simulink model "Ecm_2RC_battery"  (R2022a)
settings: Solver=FixedStepAuto  StartTime=0.0  StopTime=3600  FixedStep=0.1  RelTol=1e-3
values from neighbouring files (symbols this model uses):
  T_init = 293.15    [cell_data.mat]
libraries: fl_lib x1074, LiBatteryElements_lib x540, nesl_utility x102
(part 9 of 18)

== system Ecm_2RC_battery/Subsystem4/Subsystem4 ==
  Temp : Inport
  C1 : LiBatteryElements_lib/C_table  C_Table=C1_LUT F  SOC_Table=SOC_LUT  Temp_Table=Temperature_LUT K  v0=0 V
      settings: SourceProductBaseCode=SS  InternalSimscapePortConfiguration="{\"Bottom\":[],\"Left\":[{\"id\":\"p\",\"label\":\"+\",\"type\":\"foundation.electrical.electrical\"},{\"id\":\"T\",\"label\":\"T\",\"type\":\"input\"},{\"id\":\"SOC\",\"label\":\"SOC\",\"type\":\"input\"}],\"Right\":[{\"id\":\"n\",\"label\":\"-\",\"type\":\"foundation.electrical.electrical\"}],\"Top\":[]}"
  C2 : LiBatteryElements_lib/C_table  C_Table=C2_LUT F  SOC_Table=SOC_LUT  Temp_Table=Temperature_LUT K  v0=0 V
      settings: SourceProductBaseCode=SS  InternalSimscapePortConfiguration="{\"Bottom\":[],\"Left\":[{\"id\":\"p\",\"label\":\"+\",\"type\":\"foundation.electrical.electrical\"},{\"id\":\"T\",\"label\":\"T\",\"type\":\"input\"},{\"id\":\"SOC\",\"label\":\"SOC\",\"type\":\"input\"}],\"Right\":[{\"id\":\"n\",\"label\":\"-\",\"type\":\"foundation.electrical.electrical\"}],\"Top\":[]}"
  Controlled Temperature Source : fl_lib/Thermal/Thermal Sources/Controlled Temperature Source
      settings: SourceProductBaseCode=PW,SS,VE
  Convective Heat Transfer : fl_lib/Thermal/Thermal Elements/Convective Heat Transfer  area=cell_area m^2  heat_tr_coeff=h_conv W/(m^2 * K)  T_specify=off  T_priority=None  T=0 K  T_nominal_specify=off  T_nominal_unit=K  T_nominal_value=1  Q_specify=off  Q_priority=None  Q=0 W  Q_nominal_specify=off  Q_nominal_unit=W  Q_nominal_value=1
      settings: SourceProductBaseCode=PW,SS,VE
  Em_table : LiBatteryElements_lib/Em_table  C_Table=Capacity_LUT hr*A  Em_Table=Em_LUT V  SOC_Table=SOC_LUT  Temp_Table=Temperature_LUT K  Qinit=Qe_init hr*A
      settings: SourceProductBaseCode=SS  InternalSimscapePortConfiguration="{\"Bottom\":[],\"Left\":[{\"id\":\"p\",\"label\":\"+\",\"type\":\"foundation.electrical.electrical\"},{\"id\":\"C\",\"label\":\"C\",\"type\":\"output\"},{\"id\":\"SOC\",\"label\":\"SOC\",\"type\":\"output\"}],\"Right\":[{\"id\":\"n\",\"label\":\"-\",\"type\":\"foundation.electrical.electrical\"},{\"id\":\"T\",\"label\":\"T\",\"type\":\"input\"}],\"Top\":[]}"
  R0 : LiBatteryElements_lib/R_table  R_Table=R0_LUT Ohm  SOC_Table=SOC_LUT  Temp_Table=Temperature_LUT K
      settings: SourceProductBaseCode=SS  InternalSimscapePortConfiguration="{\"Bottom\":[],\"Left\":[{\"id\":\"p\",\"label\":\"+\",\"type\":\"foundation.electrical.electrical\"},{\"id\":\"T\",\"label\":\"T\",\"type\":\"input\"},{\"id\":\"SOC\",\"label\":\"SOC\",\"type\":\"input\"}],\"Right\":[{\"id\":\"n\",\"label\":\"-\",\"type\":\"foundation.electrical.electrical\"},{\"id\":\"pow\",\"label\":\"POW\",\"type\":\"output\"}],\"Top\":[]}"
  R1 : LiBatteryElements_lib/R_table  R_Table=R1_LUT Ohm  SOC_Table=SOC_LUT  Temp_Table=Temperature_LUT K
      settings: SourceProductBaseCode=SS  InternalSimscapePortConfiguration="{\"Bottom\":[],\"Left\":[{\"id\":\"p\",\"label\":\"+\",\"type\":\"foundation.electrical.electrical\"},{\"id\":\"T\",\"label\":\"T\",\"type\":\"input\"},{\"id\":\"SOC\",\"label\":\"SOC\",\"type\":\"input\"}],\"Right\":[{\"id\":\"n\",\"label\":\"-\",\"type\":\"foundation.electrical.electrical\"},{\"id\":\"pow\",\"label\":\"POW\",\"type\":\"output\"}],\"Top\":[]}"
  R2 : LiBatteryElements_lib/R_table  R_Table=R2_LUT Ohm  SOC_Table=SOC_LUT  Temp_Table=Temperature_LUT K
      settings: SourceProductBaseCode=SS  InternalSimscapePortConfiguration="{\"Bottom\":[],\"Left\":[{\"id\":\"p\",\"label\":\"+\",\"type\":\"foundation.electrical.electrical\"},{\"id\":\"T\",\"label\":\"T\",\"type\":\"input\"},{\"id\":\"SOC\",\"label\":\"SOC\",\"type\":\"input\"}],\"Right\":[{\"id\":\"n\",\"label\":\"-\",\"type\":\"foundation.electrical.electrical\"},{\"id\":\"pow\",\"label\":\"POW\",\"type\":\"output\"}],\"Top\":[]}"
  Simulink-PS Converter1 : nesl_utility/Simulink-PS Converter  PhysicalDomain=network_engine_domain  SubClassName=ps_input  LeftPortType=input  RightPortType=output  PseudoPeriodic=off  Frequencies=[]  NoiseDistribution=none  NoiseParameters=[]  Unit=degC  AffineConversion=on  FilteringAndDerivatives=zero  SimscapeFilterOrder=1  InputFilterTimeConstant=.001  UdotUserProvided=1
      settings: SourceProductBaseCode=SS,PW,VE
  Sum : Subsystem
      mask Display:
      | port_label('RConn',1,'+');
      | port_label('RConn',2,'+');
      | port_label('RConn',3,'+');
  Thermal Model : Subsystem
  Thermal Reference : fl_lib/Thermal/Thermal Elements/Thermal Reference
      settings: SourceProductBaseCode=PW,SS,VE
  + : PMIOPort  Side=Left
  SoC : PMIOPort  Port=2  Side=Right
  Charge : PMIOPort  Port=3  Side=Right
  - : PMIOPort  Port=4  Side=Right
  wires:
  Temp/1 -> Simulink-PS Converter1/1
  connections:
  C1/RConn1 -- R1/RConn1 -- R2/LConn1 -- C2/LConn1
  C1/LConn2 -- R0/LConn2 -- R2/LConn2 -- C2/LConn2 -- Thermal Model/RConn1 -- Em_table/RConn2 -- R1/LConn2
  R0/RConn2 -- Sum/RConn3
  R1/LConn1 -- C1/LConn1 -- Em_table/LConn1
  Convective Heat Transfer/RConn1 -- Thermal Model/LConn2
  R2/RConn1 -- R0/LConn1 -- C2/RConn1
  Sum/RConn2 -- R2/RConn2
  R1/RConn2 -- Sum/RConn1
  SoC/RConn1 -- R0/LConn3 -- C2/LConn3 -- R2/LConn3 -- Em_table/LConn3 -- C1/LConn3 -- R1/LConn3
  Sum/LConn1 -- Thermal Model/LConn1
  Controlled Temperature Source/RConn1 -- Simulink-PS Converter1/RConn1
  Thermal Reference/LConn1 -- Controlled Temperature Source/RConn2
  Controlled Temperature Source/LConn1 -- Convective Heat Transfer/LConn1
  Em_table/RConn1 -- -/RConn1
  R0/RConn1 -- +/RConn1
  Em_table/LConn2 -- Charge/RConn1

== system Ecm_2RC_battery/Subsystem4/Subsystem5 ==
  Temp : Inport
  C1 : LiBatteryElements_lib/C_table  C_Table=C1_LUT F  SOC_Table=SOC_LUT  Temp_Table=Temperature_LUT K  v0=0 V
      settings: SourceProductBaseCode=SS  InternalSimscapePortConfiguration="{\"Bottom\":[],\"Left\":[{\"id\":\"p\",\"label\":\"+\",\"type\":\"foundation.electrical.electrical\"},{\"id\":\"T\",\"label\":\"T\",\"type\":\"input\"},{\"id\":\"SOC\",\"label\":\"SOC\",\"type\":\"input\"}],\"Right\":[{\"id\":\"n\",\"label\":\"-\",\"type\":\"foundation.electrical.electrical\"}],\"Top\":[]}"
  C2 : LiBatteryElements_lib/C_table  C_Table=C2_LUT F  SOC_Table=SOC_LUT  Temp_Table=Temperature_LUT K  v0=0 V
      settings: SourceProductBaseCode=SS  InternalSimscapePortConfiguration="{\"Bottom\":[],\"Left\":[{\"id\":\"p\",\"label\":\"+\",\"type\":\"foundation.electrical.electrical\"},{\"id\":\"T\",\"label\":\"T\",\"type\":\"input\"},{\"id\":\"SOC\",\"label\":\"SOC\",\"type\":\"input\"}],\"Right\":[{\"id\":\"n\",\"label\":\"-\",\"type\":\"foundation.electrical.electrical\"}],\"Top\":[]}"
  Controlled Temperature Source : fl_lib/Thermal/Thermal Sources/Controlled Temperature Source
      settings: SourceProductBaseCode=PW,SS,VE
  Convective Heat Transfer : fl_lib/Thermal/Thermal Elements/Convective Heat Transfer  area=cell_area m^2  heat_tr_coeff=h_conv W/(m^2 * K)  T_specify=off  T_priority=None  T=0 K  T_nominal_specify=off  T_nominal_unit=K  T_nominal_value=1  Q_specify=off  Q_priority=None  Q=0 W  Q_nominal_specify=off  Q_nominal_unit=W  Q_nominal_value=1
      settings: SourceProductBaseCode=PW,SS,VE
  Em_table : LiBatteryElements_lib/Em_table  C_Table=Capacity_LUT hr*A  Em_Table=Em_LUT V  SOC_Table=SOC_LUT  Temp_Table=Temperature_LUT K  Qinit=Qe_init hr*A
      settings: SourceProductBaseCode=SS  InternalSimscapePortConfiguration="{\"Bottom\":[],\"Left\":[{\"id\":\"p\",\"label\":\"+\",\"type\":\"foundation.electrical.electrical\"},{\"id\":\"C\",\"label\":\"C\",\"type\":\"output\"},{\"id\":\"SOC\",\"label\":\"SOC\",\"type\":\"output\"}],\"Right\":[{\"id\":\"n\",\"label\":\"-\",\"type\":\"foundation.electrical.electrical\"},{\"id\":\"T\",\"label\":\"T\",\"type\":\"input\"}],\"Top\":[]}"
  R0 : LiBatteryElements_lib/R_table  R_Table=R0_LUT Ohm  SOC_Table=SOC_LUT  Temp_Table=Temperature_LUT K
      settings: SourceProductBaseCode=SS  InternalSimscapePortConfiguration="{\"Bottom\":[],\"Left\":[{\"id\":\"p\",\"label\":\"+\",\"type\":\"foundation.electrical.electrical\"},{\"id\":\"T\",\"label\":\"T\",\"type\":\"input\"},{\"id\":\"SOC\",\"label\":\"SOC\",\"type\":\"input\"}],\"Right\":[{\"id\":\"n\",\"label\":\"-\",\"type\":\"foundation.electrical.electrical\"},{\"id\":\"pow\",\"label\":\"POW\",\"type\":\"output\"}],\"Top\":[]}"
  R1 : LiBatteryElements_lib/R_table  R_Table=R1_LUT Ohm  SOC_Table=SOC_LUT  Temp_Table=Temperature_LUT K
      settings: SourceProductBaseCode=SS  InternalSimscapePortConfiguration="{\"Bottom\":[],\"Left\":[{\"id\":\"p\",\"label\":\"+\",\"type\":\"foundation.electrical.electrical\"},{\"id\":\"T\",\"label\":\"T\",\"type\":\"input\"},{\"id\":\"SOC\",\"label\":\"SOC\",\"type\":\"input\"}],\"Right\":[{\"id\":\"n\",\"label\":\"-\",\"type\":\"foundation.electrical.electrical\"},{\"id\":\"pow\",\"label\":\"POW\",\"type\":\"output\"}],\"Top\":[]}"
  R2 : LiBatteryElements_lib/R_table  R_Table=R2_LUT Ohm  SOC_Table=SOC_LUT  Temp_Table=Temperature_LUT K
      settings: SourceProductBaseCode=SS  InternalSimscapePortConfiguration="{\"Bottom\":[],\"Left\":[{\"id\":\"p\",\"label\":\"+\",\"type\":\"foundation.electrical.electrical\"},{\"id\":\"T\",\"label\":\"T\",\"type\":\"input\"},{\"id\":\"SOC\",\"label\":\"SOC\",\"type\":\"input\"}],\"Right\":[{\"id\":\"n\",\"label\":\"-\",\"type\":\"foundation.electrical.electrical\"},{\"id\":\"pow\",\"label\":\"POW\",\"type\":\"output\"}],\"Top\":[]}"
  Simulink-PS Converter1 : nesl_utility/Simulink-PS Converter  PhysicalDomain=network_engine_domain  SubClassName=ps_input  LeftPortType=input  RightPortType=output  PseudoPeriodic=off  Frequencies=[]  NoiseDistribution=none  NoiseParameters=[]  Unit=degC  AffineConversion=on  FilteringAndDerivatives=zero  SimscapeFilterOrder=1  InputFilterTimeConstant=.001  UdotUserProvided=1
      settings: SourceProductBaseCode=SS,PW,VE
  Sum : Subsystem
      mask Display:
      | port_label('RConn',1,'+');
      | port_label('RConn',2,'+');
      | port_label('RConn',3,'+');
  Thermal Model : Subsystem
  Thermal Reference : fl_lib/Thermal/Thermal Elements/Thermal Reference
      settings: SourceProductBaseCode=PW,SS,VE
  + : PMIOPort  Side=Left
  SoC : PMIOPort  Port=2  Side=Right
  Charge : PMIOPort  Port=3  Side=Right
  - : PMIOPort  Port=4  Side=Right
  wires:
  Temp/1 -> Simulink-PS Converter1/1
  connections:
  C1/RConn1 -- R1/RConn1 -- R2/LConn1 -- C2/LConn1
  C1/LConn2 -- R0/LConn2 -- R2/LConn2 -- C2/LConn2 -- Thermal Model/RConn1 -- Em_table/RConn2 -- R1/LConn2
  R0/RConn2 -- Sum/RConn3
  R1/LConn1 -- C1/LConn1 -- Em_table/LConn1
  Convective Heat Transfer/RConn1 -- Thermal Model/LConn2
  R2/RConn1 -- R0/LConn1 -- C2/RConn1
  Sum/RConn2 -- R2/RConn2
  R1/RConn2 -- Sum/RConn1
  SoC/RConn1 -- R0/LConn3 -- C2/LConn3 -- R2/LConn3 -- Em_table/LConn3 -- C1/LConn3 -- R1/LConn3
  Sum/LConn1 -- Thermal Model/LConn1
  Controlled Temperature Source/RConn1 -- Simulink-PS Converter1/RConn1
  Thermal Reference/LConn1 -- Controlled Temperature Source/RConn2
  Controlled Temperature Source/LConn1 -- Convective Heat Transfer/LConn1
  Em_table/RConn1 -- -/RConn1
  R0/RConn1 -- +/RConn1
  Em_table/LConn2 -- Charge/RConn1

== system Ecm_2RC_battery/Subsystem4/Subsystem6 ==
  Temp : Inport
  C1 : LiBatteryElements_lib/C_table  C_Table=C1_LUT F  SOC_Table=SOC_LUT  Temp_Table=Temperature_LUT K  v0=0 V
      settings: SourceProductBaseCode=SS  InternalSimscapePortConfiguration="{\"Bottom\":[],\"Left\":[{\"id\":\"p\",\"label\":\"+\",\"type\":\"foundation.electrical.electrical\"},{\"id\":\"T\",\"label\":\"T\",\"type\":\"input\"},{\"id\":\"SOC\",\"label\":\"SOC\",\"type\":\"input\"}],\"Right\":[{\"id\":\"n\",\"label\":\"-\",\"type\":\"foundation.electrical.electrical\"}],\"Top\":[]}"
  C2 : LiBatteryElements_lib/C_table  C_Table=C2_LUT F  SOC_Table=SOC_LUT  Temp_Table=Temperature_LUT K  v0=0 V
      settings: SourceProductBaseCode=SS  InternalSimscapePortConfiguration="{\"Bottom\":[],\"Left\":[{\"id\":\"p\",\"label\":\"+\",\"type\":\"foundation.electrical.electrical\"},{\"id\":\"T\",\"label\":\"T\",\"type\":\"input\"},{\"id\":\"SOC\",\"label\":\"SOC\",\"type\":\"input\"}],\"Right\":[{\"id\":\"n\",\"label\":\"-\",\"type\":\"foundation.electrical.electrical\"}],\"Top\":[]}"
  Controlled Temperature Source : fl_lib/Thermal/Thermal Sources/Controlled Temperature Source
      settings: SourceProductBaseCode=PW,SS,VE
  Convective Heat Transfer : fl_lib/Thermal/Thermal Elements/Convective Heat Transfer  area=cell_area m^2  heat_tr_coeff=h_conv W/(m^2 * K)  T_specify=off  T_priority=None  T=0 K  T_nominal_specify=off  T_nominal_unit=K  T_nominal_value=1  Q_specify=off  Q_priority=None  Q=0 W  Q_nominal_specify=off  Q_nominal_unit=W  Q_nominal_value=1
      settings: SourceProductBaseCode=PW,SS,VE
  Em_table : LiBatteryElements_lib/Em_table  C_Table=Capacity_LUT hr*A  Em_Table=Em_LUT V  SOC_Table=SOC_LUT  Temp_Table=Temperature_LUT K  Qinit=Qe_init hr*A
      settings: SourceProductBaseCode=SS  InternalSimscapePortConfiguration="{\"Bottom\":[],\"Left\":[{\"id\":\"p\",\"label\":\"+\",\"type\":\"foundation.electrical.electrical\"},{\"id\":\"C\",\"label\":\"C\",\"type\":\"output\"},{\"id\":\"SOC\",\"label\":\"SOC\",\"type\":\"output\"}],\"Right\":[{\"id\":\"n\",\"label\":\"-\",\"type\":\"foundation.electrical.electrical\"},{\"id\":\"T\",\"label\":\"T\",\"type\":\"input\"}],\"Top\":[]}"
  R0 : LiBatteryElements_lib/R_table  R_Table=R0_LUT Ohm  SOC_Table=SOC_LUT  Temp_Table=Temperature_LUT K
      settings: SourceProductBaseCode=SS  InternalSimscapePortConfiguration="{\"Bottom\":[],\"Left\":[{\"id\":\"p\",\"label\":\"+\",\"type\":\"foundation.electrical.electrical\"},{\"id\":\"T\",\"label\":\"T\",\"type\":\"input\"},{\"id\":\"SOC\",\"label\":\"SOC\",\"type\":\"input\"}],\"Right\":[{\"id\":\"n\",\"label\":\"-\",\"type\":\"foundation.electrical.electrical\"},{\"id\":\"pow\",\"label\":\"POW\",\"type\":\"output\"}],\"Top\":[]}"
  R1 : LiBatteryElements_lib/R_table  R_Table=R1_LUT Ohm  SOC_Table=SOC_LUT  Temp_Table=Temperature_LUT K
      settings: SourceProductBaseCode=SS  InternalSimscapePortConfiguration="{\"Bottom\":[],\"Left\":[{\"id\":\"p\",\"label\":\"+\",\"type\":\"foundation.electrical.electrical\"},{\"id\":\"T\",\"label\":\"T\",\"type\":\"input\"},{\"id\":\"SOC\",\"label\":\"SOC\",\"type\":\"input\"}],\"Right\":[{\"id\":\"n\",\"label\":\"-\",\"type\":\"foundation.electrical.electrical\"},{\"id\":\"pow\",\"label\":\"POW\",\"type\":\"output\"}],\"Top\":[]}"
  R2 : LiBatteryElements_lib/R_table  R_Table=R2_LUT Ohm  SOC_Table=SOC_LUT  Temp_Table=Temperature_LUT K
      settings: SourceProductBaseCode=SS  InternalSimscapePortConfiguration="{\"Bottom\":[],\"Left\":[{\"id\":\"p\",\"label\":\"+\",\"type\":\"foundation.electrical.electrical\"},{\"id\":\"T\",\"label\":\"T\",\"type\":\"input\"},{\"id\":\"SOC\",\"label\":\"SOC\",\"type\":\"input\"}],\"Right\":[{\"id\":\"n\",\"label\":\"-\",\"type\":\"foundation.electrical.electrical\"},{\"id\":\"pow\",\"label\":\"POW\",\"type\":\"output\"}],\"Top\":[]}"
  Simulink-PS Converter1 : nesl_utility/Simulink-PS Converter  PhysicalDomain=network_engine_domain  SubClassName=ps_input  LeftPortType=input  RightPortType=output  PseudoPeriodic=off  Frequencies=[]  NoiseDistribution=none  NoiseParameters=[]  Unit=degC  AffineConversion=on  FilteringAndDerivatives=zero  SimscapeFilterOrder=1  InputFilterTimeConstant=.001  UdotUserProvided=1
      settings: SourceProductBaseCode=SS,PW,VE
  Sum : Subsystem
      mask Display:
      | port_label('RConn',1,'+');
      | port_label('RConn',2,'+');
      | port_label('RConn',3,'+');
  Thermal Model : Subsystem
  Thermal Reference : fl_lib/Thermal/Thermal Elements/Thermal Reference
      settings: SourceProductBaseCode=PW,SS,VE
  + : PMIOPort  Side=Left
  SoC : PMIOPort  Port=2  Side=Right
  Charge : PMIOPort  Port=3  Side=Right
  - : PMIOPort  Port=4  Side=Right
  wires:
  Temp/1 -> Simulink-PS Converter1/1
  connections:
  C1/RConn1 -- R1/RConn1 -- R2/LConn1 -- C2/LConn1
  C1/LConn2 -- R0/LConn2 -- R2/LConn2 -- C2/LConn2 -- Thermal Model/RConn1 -- Em_table/RConn2 -- R1/LConn2
  R0/RConn2 -- Sum/RConn3
  R1/LConn1 -- C1/LConn1 -- Em_table/LConn1
  Convective Heat Transfer/RConn1 -- Thermal Model/LConn2
  R2/RConn1 -- R0/LConn1 -- C2/RConn1
  Sum/RConn2 -- R2/RConn2
  R1/RConn2 -- Sum/RConn1
  SoC/RConn1 -- R0/LConn3 -- C2/LConn3 -- R2/LConn3 -- Em_table/LConn3 -- C1/LConn3 -- R1/LConn3
  Sum/LConn1 -- Thermal Model/LConn1
  Controlled Temperature Source/RConn1 -- Simulink-PS Converter1/RConn1
  Thermal Reference/LConn1 -- Controlled Temperature Source/RConn2
  Controlled Temperature Source/LConn1 -- Convective Heat Transfer/LConn1
  Em_table/RConn1 -- -/RConn1
  R0/RConn1 -- +/RConn1
  Em_table/LConn2 -- Charge/RConn1

== system Ecm_2RC_battery/Subsystem4/Subsystem7 ==
  Temp : Inport
  C1 : LiBatteryElements_lib/C_table  C_Table=C1_LUT F  SOC_Table=SOC_LUT  Temp_Table=Temperature_LUT K  v0=0 V
      settings: SourceProductBaseCode=SS  InternalSimscapePortConfiguration="{\"Bottom\":[],\"Left\":[{\"id\":\"p\",\"label\":\"+\",\"type\":\"foundation.electrical.electrical\"},{\"id\":\"T\",\"label\":\"T\",\"type\":\"input\"},{\"id\":\"SOC\",\"label\":\"SOC\",\"type\":\"input\"}],\"Right\":[{\"id\":\"n\",\"label\":\"-\",\"type\":\"foundation.electrical.electrical\"}],\"Top\":[]}"
  C2 : LiBatteryElements_lib/C_table  C_Table=C2_LUT F  SOC_Table=SOC_LUT  Temp_Table=Temperature_LUT K  v0=0 V
      settings: SourceProductBaseCode=SS  InternalSimscapePortConfiguration="{\"Bottom\":[],\"Left\":[{\"id\":\"p\",\"label\":\"+\",\"type\":\"foundation.electrical.electrical\"},{\"id\":\"T\",\"label\":\"T\",\"type\":\"input\"},{\"id\":\"SOC\",\"label\":\"SOC\",\"type\":\"input\"}],\"Right\":[{\"id\":\"n\",\"label\":\"-\",\"type\":\"foundation.electrical.electrical\"}],\"Top\":[]}"
  Controlled Temperature Source : fl_lib/Thermal/Thermal Sources/Controlled Temperature Source
      settings: SourceProductBaseCode=PW,SS,VE
  Convective Heat Transfer : fl_lib/Thermal/Thermal Elements/Convective Heat Transfer  area=cell_area m^2  heat_tr_coeff=h_conv W/(m^2 * K)  T_specify=off  T_priority=None  T=0 K  T_nominal_specify=off  T_nominal_unit=K  T_nominal_value=1  Q_specify=off  Q_priority=None  Q=0 W  Q_nominal_specify=off  Q_nominal_unit=W  Q_nominal_value=1
      settings: SourceProductBaseCode=PW,SS,VE
  Em_table : LiBatteryElements_lib/Em_table  C_Table=Capacity_LUT hr*A  Em_Table=Em_LUT V  SOC_Table=SOC_LUT  Temp_Table=Temperature_LUT K  Qinit=Qe_init hr*A
      settings: SourceProductBaseCode=SS  InternalSimscapePortConfiguration="{\"Bottom\":[],\"Left\":[{\"id\":\"p\",\"label\":\"+\",\"type\":\"foundation.electrical.electrical\"},{\"id\":\"C\",\"label\":\"C\",\"type\":\"output\"},{\"id\":\"SOC\",\"label\":\"SOC\",\"type\":\"output\"}],\"Right\":[{\"id\":\"n\",\"label\":\"-\",\"type\":\"foundation.electrical.electrical\"},{\"id\":\"T\",\"label\":\"T\",\"type\":\"input\"}],\"Top\":[]}"
  R0 : LiBatteryElements_lib/R_table  R_Table=R0_LUT Ohm  SOC_Table=SOC_LUT  Temp_Table=Temperature_LUT K
      settings: SourceProductBaseCode=SS  InternalSimscapePortConfiguration="{\"Bottom\":[],\"Left\":[{\"id\":\"p\",\"label\":\"+\",\"type\":\"foundation.electrical.electrical\"},{\"id\":\"T\",\"label\":\"T\",\"type\":\"input\"},{\"id\":\"SOC\",\"label\":\"SOC\",\"type\":\"input\"}],\"Right\":[{\"id\":\"n\",\"label\":\"-\",\"type\":\"foundation.electrical.electrical\"},{\"id\":\"pow\",\"label\":\"POW\",\"type\":\"output\"}],\"Top\":[]}"
  R1 : LiBatteryElements_lib/R_table  R_Table=R1_LUT Ohm  SOC_Table=SOC_LUT  Temp_Table=Temperature_LUT K
      settings: SourceProductBaseCode=SS  InternalSimscapePortConfiguration="{\"Bottom\":[],\"Left\":[{\"id\":\"p\",\"label\":\"+\",\"type\":\"foundation.electrical.electrical\"},{\"id\":\"T\",\"label\":\"T\",\"type\":\"input\"},{\"id\":\"SOC\",\"label\":\"SOC\",\"type\":\"input\"}],\"Right\":[{\"id\":\"n\",\"label\":\"-\",\"type\":\"foundation.electrical.electrical\"},{\"id\":\"pow\",\"label\":\"POW\",\"type\":\"output\"}],\"Top\":[]}"
  R2 : LiBatteryElements_lib/R_table  R_Table=R2_LUT Ohm  SOC_Table=SOC_LUT  Temp_Table=Temperature_LUT K
      settings: SourceProductBaseCode=SS  InternalSimscapePortConfiguration="{\"Bottom\":[],\"Left\":[{\"id\":\"p\",\"label\":\"+\",\"type\":\"foundation.electrical.electrical\"},{\"id\":\"T\",\"label\":\"T\",\"type\":\"input\"},{\"id\":\"SOC\",\"label\":\"SOC\",\"type\":\"input\"}],\"Right\":[{\"id\":\"n\",\"label\":\"-\",\"type\":\"foundation.electrical.electrical\"},{\"id\":\"pow\",\"label\":\"POW\",\"type\":\"output\"}],\"Top\":[]}"
  Simulink-PS Converter1 : nesl_utility/Simulink-PS Converter  PhysicalDomain=network_engine_domain  SubClassName=ps_input  LeftPortType=input  RightPortType=output  PseudoPeriodic=off  Frequencies=[]  NoiseDistribution=none  NoiseParameters=[]  Unit=degC  AffineConversion=on  FilteringAndDerivatives=zero  SimscapeFilterOrder=1  InputFilterTimeConstant=.001  UdotUserProvided=1
      settings: SourceProductBaseCode=SS,PW,VE
  Sum : Subsystem
      mask Display:
      | port_label('RConn',1,'+');
      | port_label('RConn',2,'+');
      | port_label('RConn',3,'+');
  Thermal Model : Subsystem
  Thermal Reference : fl_lib/Thermal/Thermal Elements/Thermal Reference
      settings: SourceProductBaseCode=PW,SS,VE
  + : PMIOPort  Side=Left
  SoC : PMIOPort  Port=2  Side=Right
  Charge : PMIOPort  Port=3  Side=Right
  - : PMIOPort  Port=4  Side=Right
  wires:
  Temp/1 -> Simulink-PS Converter1/1
  connections:
  C1/RConn1 -- R1/RConn1 -- R2/LConn1 -- C2/LConn1
  C1/LConn2 -- R0/LConn2 -- R2/LConn2 -- C2/LConn2 -- Thermal Model/RConn1 -- Em_table/RConn2 -- R1/LConn2
  R0/RConn2 -- Sum/RConn3
  R1/LConn1 -- C1/LConn1 -- Em_table/LConn1
  Convective Heat Transfer/RConn1 -- Thermal Model/LConn2
  R2/RConn1 -- R0/LConn1 -- C2/RConn1
  Sum/RConn2 -- R2/RConn2
  R1/RConn2 -- Sum/RConn1
  SoC/RConn1 -- R0/LConn3 -- C2/LConn3 -- R2/LConn3 -- Em_table/LConn3 -- C1/LConn3 -- R1/LConn3
  Sum/LConn1 -- Thermal Model/LConn1
  Controlled Temperature Source/RConn1 -- Simulink-PS Converter1/RConn1
  Thermal Reference/LConn1 -- Controlled Temperature Source/RConn2
  Controlled Temperature Source/LConn1 -- Convective Heat Transfer/LConn1
  Em_table/RConn1 -- -/RConn1
  R0/RConn1 -- +/RConn1
  Em_table/LConn2 -- Charge/RConn1

== system Ecm_2RC_battery/Subsystem4/Subsystem8 ==
  Temp : Inport
  C1 : LiBatteryElements_lib/C_table  C_Table=C1_LUT F  SOC_Table=SOC_LUT  Temp_Table=Temperature_LUT K  v0=0 V
      settings: SourceProductBaseCode=SS  InternalSimscapePortConfiguration="{\"Bottom\":[],\"Left\":[{\"id\":\"p\",\"label\":\"+\",\"type\":\"foundation.electrical.electrical\"},{\"id\":\"T\",\"label\":\"T\",\"type\":\"input\"},{\"id\":\"SOC\",\"label\":\"SOC\",\"type\":\"input\"}],\"Right\":[{\"id\":\"n\",\"label\":\"-\",\"type\":\"foundation.electrical.electrical\"}],\"Top\":[]}"
  C2 : LiBatteryElements_lib/C_table  C_Table=C2_LUT F  SOC_Table=SOC_LUT  Temp_Table=Temperature_LUT K  v0=0 V
      settings: SourceProductBaseCode=SS  InternalSimscapePortConfiguration="{\"Bottom\":[],\"Left\":[{\"id\":\"p\",\"label\":\"+\",\"type\":\"foundation.electrical.electrical\"},{\"id\":\"T\",\"label\":\"T\",\"type\":\"input\"},{\"id\":\"SOC\",\"label\":\"SOC\",\"type\":\"input\"}],\"Right\":[{\"id\":\"n\",\"label\":\"-\",\"type\":\"foundation.electrical.electrical\"}],\"Top\":[]}"
  Controlled Temperature Source : fl_lib/Thermal/Thermal Sources/Controlled Temperature Source
      settings: SourceProductBaseCode=PW,SS,VE
  Convective Heat Transfer : fl_lib/Thermal/Thermal Elements/Convective Heat Transfer  area=cell_area m^2  heat_tr_coeff=h_conv W/(m^2 * K)  T_specify=off  T_priority=None  T=0 K  T_nominal_specify=off  T_nominal_unit=K  T_nominal_value=1  Q_specify=off  Q_priority=None  Q=0 W  Q_nominal_specify=off  Q_nominal_unit=W  Q_nominal_value=1
      settings: SourceProductBaseCode=PW,SS,VE
  Em_table : LiBatteryElements_lib/Em_table  C_Table=Capacity_LUT hr*A  Em_Table=Em_LUT V  SOC_Table=SOC_LUT  Temp_Table=Temperature_LUT K  Qinit=Qe_init hr*A
      settings: SourceProductBaseCode=SS  InternalSimscapePortConfiguration="{\"Bottom\":[],\"Left\":[{\"id\":\"p\",\"label\":\"+\",\"type\":\"foundation.electrical.electrical\"},{\"id\":\"C\",\"label\":\"C\",\"type\":\"output\"},{\"id\":\"SOC\",\"label\":\"SOC\",\"type\":\"output\"}],\"Right\":[{\"id\":\"n\",\"label\":\"-\",\"type\":\"foundation.electrical.electrical\"},{\"id\":\"T\",\"label\":\"T\",\"type\":\"input\"}],\"Top\":[]}"
  R0 : LiBatteryElements_lib/R_table  R_Table=R0_LUT Ohm  SOC_Table=SOC_LUT  Temp_Table=Temperature_LUT K
      settings: SourceProductBaseCode=SS  InternalSimscapePortConfiguration="{\"Bottom\":[],\"Left\":[{\"id\":\"p\",\"label\":\"+\",\"type\":\"foundation.electrical.electrical\"},{\"id\":\"T\",\"label\":\"T\",\"type\":\"input\"},{\"id\":\"SOC\",\"label\":\"SOC\",\"type\":\"input\"}],\"Right\":[{\"id\":\"n\",\"label\":\"-\",\"type\":\"foundation.electrical.electrical\"},{\"id\":\"pow\",\"label\":\"POW\",\"type\":\"output\"}],\"Top\":[]}"
  R1 : LiBatteryElements_lib/R_table  R_Table=R1_LUT Ohm  SOC_Table=SOC_LUT  Temp_Table=Temperature_LUT K
      settings: SourceProductBaseCode=SS  InternalSimscapePortConfiguration="{\"Bottom\":[],\"Left\":[{\"id\":\"p\",\"label\":\"+\",\"type\":\"foundation.electrical.electrical\"},{\"id\":\"T\",\"label\":\"T\",\"type\":\"input\"},{\"id\":\"SOC\",\"label\":\"SOC\",\"type\":\"input\"}],\"Right\":[{\"id\":\"n\",\"label\":\"-\",\"type\":\"foundation.electrical.electrical\"},{\"id\":\"pow\",\"label\":\"POW\",\"type\":\"output\"}],\"Top\":[]}"
  R2 : LiBatteryElements_lib/R_table  R_Table=R2_LUT Ohm  SOC_Table=SOC_LUT  Temp_Table=Temperature_LUT K
      settings: SourceProductBaseCode=SS  InternalSimscapePortConfiguration="{\"Bottom\":[],\"Left\":[{\"id\":\"p\",\"label\":\"+\",\"type\":\"foundation.electrical.electrical\"},{\"id\":\"T\",\"label\":\"T\",\"type\":\"input\"},{\"id\":\"SOC\",\"label\":\"SOC\",\"type\":\"input\"}],\"Right\":[{\"id\":\"n\",\"label\":\"-\",\"type\":\"foundation.electrical.electrical\"},{\"id\":\"pow\",\"label\":\"POW\",\"type\":\"output\"}],\"Top\":[]}"
  Simulink-PS Converter1 : nesl_utility/Simulink-PS Converter  PhysicalDomain=network_engine_domain  SubClassName=ps_input  LeftPortType=input  RightPortType=output  PseudoPeriodic=off  Frequencies=[]  NoiseDistribution=none  NoiseParameters=[]  Unit=degC  AffineConversion=on  FilteringAndDerivatives=zero  SimscapeFilterOrder=1  InputFilterTimeConstant=.001  UdotUserProvided=1
      settings: SourceProductBaseCode=SS,PW,VE
  Sum : Subsystem
      mask Display:
      | port_label('RConn',1,'+');
      | port_label('RConn',2,'+');
      | port_label('RConn',3,'+');
  Thermal Model : Subsystem
  Thermal Reference : fl_lib/Thermal/Thermal Elements/Thermal Reference
      settings: SourceProductBaseCode=PW,SS,VE
  + : PMIOPort  Side=Left
  SoC : PMIOPort  Port=2  Side=Right
  Charge : PMIOPort  Port=3  Side=Right
  - : PMIOPort  Port=4  Side=Right
  wires:
  Temp/1 -> Simulink-PS Converter1/1
  connections:
  C1/RConn1 -- R1/RConn1 -- R2/LConn1 -- C2/LConn1
  C1/LConn2 -- R0/LConn2 -- R2/LConn2 -- C2/LConn2 -- Thermal Model/RConn1 -- Em_table/RConn2 -- R1/LConn2
  R0/RConn2 -- Sum/RConn3
  R1/LConn1 -- C1/LConn1 -- Em_table/LConn1
  Convective Heat Transfer/RConn1 -- Thermal Model/LConn2
  R2/RConn1 -- R0/LConn1 -- C2/RConn1
  Sum/RConn2 -- R2/RConn2
  R1/RConn2 -- Sum/RConn1
  SoC/RConn1 -- R0/LConn3 -- C2/LConn3 -- R2/LConn3 -- Em_table/LConn3 -- C1/LConn3 -- R1/LConn3
  Sum/LConn1 -- Thermal Model/LConn1
  Controlled Temperature Source/RConn1 -- Simulink-PS Converter1/RConn1
  Thermal Reference/LConn1 -- Controlled Temperature Source/RConn2
  Controlled Temperature Source/LConn1 -- Convective Heat Transfer/LConn1
  Em_table/RConn1 -- -/RConn1
  R0/RConn1 -- +/RConn1
  Em_table/LConn2 -- Charge/RConn1

== system Ecm_2RC_battery/Subsystem4/Subsystem9 ==
  Temp : Inport
  C1 : LiBatteryElements_lib/C_table  C_Table=C1_LUT F  SOC_Table=SOC_LUT  Temp_Table=Temperature_LUT K  v0=0 V
      settings: SourceProductBaseCode=SS  InternalSimscapePortConfiguration="{\"Bottom\":[],\"Left\":[{\"id\":\"p\",\"label\":\"+\",\"type\":\"foundation.electrical.electrical\"},{\"id\":\"T\",\"label\":\"T\",\"type\":\"input\"},{\"id\":\"SOC\",\"label\":\"SOC\",\"type\":\"input\"}],\"Right\":[{\"id\":\"n\",\"label\":\"-\",\"type\":\"foundation.electrical.electrical\"}],\"Top\":[]}"
  C2 : LiBatteryElements_lib/C_table  C_Table=C2_LUT F  SOC_Table=SOC_LUT  Temp_Table=Temperature_LUT K  v0=0 V
      settings: SourceProductBaseCode=SS  InternalSimscapePortConfiguration="{\"Bottom\":[],\"Left\":[{\"id\":\"p\",\"label\":\"+\",\"type\":\"foundation.electrical.electrical\"},{\"id\":\"T\",\"label\":\"T\",\"type\":\"input\"},{\"id\":\"SOC\",\"label\":\"SOC\",\"type\":\"input\"}],\"Right\":[{\"id\":\"n\",\"label\":\"-\",\"type\":\"foundation.electrical.electrical\"}],\"Top\":[]}"
  Controlled Temperature Source : fl_lib/Thermal/Thermal Sources/Controlled Temperature Source
      settings: SourceProductBaseCode=PW,SS,VE
  Convective Heat Transfer : fl_lib/Thermal/Thermal Elements/Convective Heat Transfer  area=cell_area m^2  heat_tr_coeff=h_conv W/(m^2 * K)  T_specify=off  T_priority=None  T=0 K  T_nominal_specify=off  T_nominal_unit=K  T_nominal_value=1  Q_specify=off  Q_priority=None  Q=0 W  Q_nominal_specify=off  Q_nominal_unit=W  Q_nominal_value=1
      settings: SourceProductBaseCode=PW,SS,VE
  Em_table : LiBatteryElements_lib/Em_table  C_Table=Capacity_LUT hr*A  Em_Table=Em_LUT V  SOC_Table=SOC_LUT  Temp_Table=Temperature_LUT K  Qinit=Qe_init hr*A
      settings: SourceProductBaseCode=SS  InternalSimscapePortConfiguration="{\"Bottom\":[],\"Left\":[{\"id\":\"p\",\"label\":\"+\",\"type\":\"foundation.electrical.electrical\"},{\"id\":\"C\",\"label\":\"C\",\"type\":\"output\"},{\"id\":\"SOC\",\"label\":\"SOC\",\"type\":\"output\"}],\"Right\":[{\"id\":\"n\",\"label\":\"-\",\"type\":\"foundation.electrical.electrical\"},{\"id\":\"T\",\"label\":\"T\",\"type\":\"input\"}],\"Top\":[]}"
  R0 : LiBatteryElements_lib/R_table  R_Table=R0_LUT Ohm  SOC_Table=SOC_LUT  Temp_Table=Temperature_LUT K
      settings: SourceProductBaseCode=SS  InternalSimscapePortConfiguration="{\"Bottom\":[],\"Left\":[{\"id\":\"p\",\"label\":\"+\",\"type\":\"foundation.electrical.electrical\"},{\"id\":\"T\",\"label\":\"T\",\"type\":\"input\"},{\"id\":\"SOC\",\"label\":\"SOC\",\"type\":\"input\"}],\"Right\":[{\"id\":\"n\",\"label\":\"-\",\"type\":\"foundation.electrical.electrical\"},{\"id\":\"pow\",\"label\":\"POW\",\"type\":\"output\"}],\"Top\":[]}"
  R1 : LiBatteryElements_lib/R_table  R_Table=R1_LUT Ohm  SOC_Table=SOC_LUT  Temp_Table=Temperature_LUT K
      settings: SourceProductBaseCode=SS  InternalSimscapePortConfiguration="{\"Bottom\":[],\"Left\":[{\"id\":\"p\",\"label\":\"+\",\"type\":\"foundation.electrical.electrical\"},{\"id\":\"T\",\"label\":\"T\",\"type\":\"input\"},{\"id\":\"SOC\",\"label\":\"SOC\",\"type\":\"input\"}],\"Right\":[{\"id\":\"n\",\"label\":\"-\",\"type\":\"foundation.electrical.electrical\"},{\"id\":\"pow\",\"label\":\"POW\",\"type\":\"output\"}],\"Top\":[]}"
  R2 : LiBatteryElements_lib/R_table  R_Table=R2_LUT Ohm  SOC_Table=SOC_LUT  Temp_Table=Temperature_LUT K
      settings: SourceProductBaseCode=SS  InternalSimscapePortConfiguration="{\"Bottom\":[],\"Left\":[{\"id\":\"p\",\"label\":\"+\",\"type\":\"foundation.electrical.electrical\"},{\"id\":\"T\",\"label\":\"T\",\"type\":\"input\"},{\"id\":\"SOC\",\"label\":\"SOC\",\"type\":\"input\"}],\"Right\":[{\"id\":\"n\",\"label\":\"-\",\"type\":\"foundation.electrical.electrical\"},{\"id\":\"pow\",\"label\":\"POW\",\"type\":\"output\"}],\"Top\":[]}"
  Simulink-PS Converter1 : nesl_utility/Simulink-PS Converter  PhysicalDomain=network_engine_domain  SubClassName=ps_input  LeftPortType=input  RightPortType=output  PseudoPeriodic=off  Frequencies=[]  NoiseDistribution=none  NoiseParameters=[]  Unit=degC  AffineConversion=on  FilteringAndDerivatives=zero  SimscapeFilterOrder=1  InputFilterTimeConstant=.001  UdotUserProvided=1
      settings: SourceProductBaseCode=SS,PW,VE
  Sum : Subsystem
      mask Display:
      | port_label('RConn',1,'+');
      | port_label('RConn',2,'+');
      | port_label('RConn',3,'+');
  Thermal Model : Subsystem
  Thermal Reference : fl_lib/Thermal/Thermal Elements/Thermal Reference
      settings: SourceProductBaseCode=PW,SS,VE
  + : PMIOPort  Side=Left
  SoC : PMIOPort  Port=2  Side=Right
  Charge : PMIOPort  Port=3  Side=Right
  - : PMIOPort  Port=4  Side=Right
  wires:
  Temp/1 -> Simulink-PS Converter1/1
  connections:
  C1/RConn1 -- R1/RConn1 -- R2/LConn1 -- C2/LConn1
  C1/LConn2 -- R0/LConn2 -- R2/LConn2 -- C2/LConn2 -- Thermal Model/RConn1 -- Em_table/RConn2 -- R1/LConn2
  R0/RConn2 -- Sum/RConn3
  R1/LConn1 -- C1/LConn1 -- Em_table/LConn1
  Convective Heat Transfer/RConn1 -- Thermal Model/LConn2
  R2/RConn1 -- R0/LConn1 -- C2/RConn1
  Sum/RConn2 -- R2/RConn2
  R1/RConn2 -- Sum/RConn1
  SoC/RConn1 -- R0/LConn3 -- C2/LConn3 -- R2/LConn3 -- Em_table/LConn3 -- C1/LConn3 -- R1/LConn3
  Sum/LConn1 -- Thermal Model/LConn1
  Controlled Temperature Source/RConn1 -- Simulink-PS Converter1/RConn1
  Thermal Reference/LConn1 -- Controlled Temperature Source/RConn2
  Controlled Temperature Source/LConn1 -- Convective Heat Transfer/LConn1
  Em_table/RConn1 -- -/RConn1
  R0/RConn1 -- +/RConn1
  Em_table/LConn2 -- Charge/RConn1

== system Ecm_2RC_battery/Subsystem5/Subsystem ==
  Temp : Inport
  C1 : LiBatteryElements_lib/C_table  C_Table=C1_LUT F  SOC_Table=SOC_LUT  Temp_Table=Temperature_LUT K  v0=0 V
      settings: SourceProductBaseCode=SS  InternalSimscapePortConfiguration="{\"Bottom\":[],\"Left\":[{\"id\":\"p\",\"label\":\"+\",\"type\":\"foundation.electrical.electrical\"},{\"id\":\"T\",\"label\":\"T\",\"type\":\"input\"},{\"id\":\"SOC\",\"label\":\"SOC\",\"type\":\"input\"}],\"Right\":[{\"id\":\"n\",\"label\":\"-\",\"type\":\"foundation.electrical.electrical\"}],\"Top\":[]}"
  C2 : LiBatteryElements_lib/C_table  C_Table=C2_LUT F  SOC_Table=SOC_LUT  Temp_Table=Temperature_LUT K  v0=0 V
      settings: SourceProductBaseCode=SS  InternalSimscapePortConfiguration="{\"Bottom\":[],\"Left\":[{\"id\":\"p\",\"label\":\"+\",\"type\":\"foundation.electrical.electrical\"},{\"id\":\"T\",\"label\":\"T\",\"type\":\"input\"},{\"id\":\"SOC\",\"label\":\"SOC\",\"type\":\"input\"}],\"Right\":[{\"id\":\"n\",\"label\":\"-\",\"type\":\"foundation.electrical.electrical\"}],\"Top\":[]}"
  Controlled Temperature Source : fl_lib/Thermal/Thermal Sources/Controlled Temperature Source
      settings: SourceProductBaseCode=PW,SS,VE
  Convective Heat Transfer : fl_lib/Thermal/Thermal Elements/Convective Heat Transfer  area=cell_area m^2  heat_tr_coeff=h_conv W/(m^2 * K)  T_specify=off  T_priority=None  T=0 K  T_nominal_specify=off  T_nominal_unit=K  T_nominal_value=1  Q_specify=off  Q_priority=None  Q=0 W  Q_nominal_specify=off  Q_nominal_unit=W  Q_nominal_value=1
      settings: SourceProductBaseCode=PW,SS,VE
  Em_table : LiBatteryElements_lib/Em_table  C_Table=Capacity_LUT hr*A  Em_Table=Em_LUT V  SOC_Table=SOC_LUT  Temp_Table=Temperature_LUT K  Qinit=Qe_init hr*A
      settings: SourceProductBaseCode=SS  InternalSimscapePortConfiguration="{\"Bottom\":[],\"Left\":[{\"id\":\"p\",\"label\":\"+\",\"type\":\"foundation.electrical.electrical\"},{\"id\":\"C\",\"label\":\"C\",\"type\":\"output\"},{\"id\":\"SOC\",\"label\":\"SOC\",\"type\":\"output\"}],\"Right\":[{\"id\":\"n\",\"label\":\"-\",\"type\":\"foundation.electrical.electrical\"},{\"id\":\"T\",\"label\":\"T\",\"type\":\"input\"}],\"Top\":[]}"
  R0 : LiBatteryElements_lib/R_table  R_Table=R0_LUT Ohm  SOC_Table=SOC_LUT  Temp_Table=Temperature_LUT K
      settings: SourceProductBaseCode=SS  InternalSimscapePortConfiguration="{\"Bottom\":[],\"Left\":[{\"id\":\"p\",\"label\":\"+\",\"type\":\"foundation.electrical.electrical\"},{\"id\":\"T\",\"label\":\"T\",\"type\":\"input\"},{\"id\":\"SOC\",\"label\":\"SOC\",\"type\":\"input\"}],\"Right\":[{\"id\":\"n\",\"label\":\"-\",\"type\":\"foundation.electrical.electrical\"},{\"id\":\"pow\",\"label\":\"POW\",\"type\":\"output\"}],\"Top\":[]}"
  R1 : LiBatteryElements_lib/R_table  R_Table=R1_LUT Ohm  SOC_Table=SOC_LUT  Temp_Table=Temperature_LUT K
      settings: SourceProductBaseCode=SS  InternalSimscapePortConfiguration="{\"Bottom\":[],\"Left\":[{\"id\":\"p\",\"label\":\"+\",\"type\":\"foundation.electrical.electrical\"},{\"id\":\"T\",\"label\":\"T\",\"type\":\"input\"},{\"id\":\"SOC\",\"label\":\"SOC\",\"type\":\"input\"}],\"Right\":[{\"id\":\"n\",\"label\":\"-\",\"type\":\"foundation.electrical.electrical\"},{\"id\":\"pow\",\"label\":\"POW\",\"type\":\"output\"}],\"Top\":[]}"
  R2 : LiBatteryElements_lib/R_table  R_Table=R2_LUT Ohm  SOC_Table=SOC_LUT  Temp_Table=Temperature_LUT K
      settings: SourceProductBaseCode=SS  InternalSimscapePortConfiguration="{\"Bottom\":[],\"Left\":[{\"id\":\"p\",\"label\":\"+\",\"type\":\"foundation.electrical.electrical\"},{\"id\":\"T\",\"label\":\"T\",\"type\":\"input\"},{\"id\":\"SOC\",\"label\":\"SOC\",\"type\":\"input\"}],\"Right\":[{\"id\":\"n\",\"label\":\"-\",\"type\":\"foundation.electrical.electrical\"},{\"id\":\"pow\",\"label\":\"POW\",\"type\":\"output\"}],\"Top\":[]}"
  Simulink-PS Converter1 : nesl_utility/Simulink-PS Converter  PhysicalDomain=network_engine_domain  SubClassName=ps_input  LeftPortType=input  RightPortType=output  PseudoPeriodic=off  Frequencies=[]  NoiseDistribution=none  NoiseParameters=[]  Unit=degC  AffineConversion=on  FilteringAndDerivatives=zero  SimscapeFilterOrder=1  InputFilterTimeConstant=.001  UdotUserProvided=1
      settings: SourceProductBaseCode=SS,PW,VE
  Sum : Subsystem
      mask Display:
      | port_label('RConn',1,'+');
      | port_label('RConn',2,'+');
      | port_label('RConn',3,'+');
  Thermal Model : Subsystem
  Thermal Reference : fl_lib/Thermal/Thermal Elements/Thermal Reference
      settings: SourceProductBaseCode=PW,SS,VE
  + : PMIOPort  Side=Left
  SoC : PMIOPort  Port=2  Side=Right
  Charge : PMIOPort  Port=3  Side=Right
  - : PMIOPort  Port=4  Side=Right
  wires:
  Temp/1 -> Simulink-PS Converter1/1
  connections:
  C1/RConn1 -- R1/RConn1 -- R2/LConn1 -- C2/LConn1
  C1/LConn2 -- R0/LConn2 -- R2/LConn2 -- C2/LConn2 -- Thermal Model/RConn1 -- Em_table/RConn2 -- R1/LConn2
  R0/RConn2 -- Sum/RConn3
  R1/LConn1 -- C1/LConn1 -- Em_table/LConn1
  Convective Heat Transfer/RConn1 -- Thermal Model/LConn2
  R2/RConn1 -- R0/LConn1 -- C2/RConn1
  Sum/RConn2 -- R2/RConn2
  R1/RConn2 -- Sum/RConn1
  SoC/RConn1 -- R0/LConn3 -- C2/LConn3 -- R2/LConn3 -- Em_table/LConn3 -- C1/LConn3 -- R1/LConn3
  Sum/LConn1 -- Thermal Model/LConn1
  Controlled Temperature Source/RConn1 -- Simulink-PS Converter1/RConn1
  Thermal Reference/LConn1 -- Controlled Temperature Source/RConn2
  Controlled Temperature Source/LConn1 -- Convective Heat Transfer/LConn1
  Em_table/RConn1 -- -/RConn1
  R0/RConn1 -- +/RConn1
  Em_table/LConn2 -- Charge/RConn1

== system Ecm_2RC_battery/Subsystem5/Subsystem1 ==
  Temp : Inport
  C1 : LiBatteryElements_lib/C_table  C_Table=C1_LUT F  SOC_Table=SOC_LUT  Temp_Table=Temperature_LUT K  v0=0 V
      settings: SourceProductBaseCode=SS  InternalSimscapePortConfiguration="{\"Bottom\":[],\"Left\":[{\"id\":\"p\",\"label\":\"+\",\"type\":\"foundation.electrical.electrical\"},{\"id\":\"T\",\"label\":\"T\",\"type\":\"input\"},{\"id\":\"SOC\",\"label\":\"SOC\",\"type\":\"input\"}],\"Right\":[{\"id\":\"n\",\"label\":\"-\",\"type\":\"foundation.electrical.electrical\"}],\"Top\":[]}"
  C2 : LiBatteryElements_lib/C_table  C_Table=C2_LUT F  SOC_Table=SOC_LUT  Temp_Table=Temperature_LUT K  v0=0 V
      settings: SourceProductBaseCode=SS  InternalSimscapePortConfiguration="{\"Bottom\":[],\"Left\":[{\"id\":\"p\",\"label\":\"+\",\"type\":\"foundation.electrical.electrical\"},{\"id\":\"T\",\"label\":\"T\",\"type\":\"input\"},{\"id\":\"SOC\",\"label\":\"SOC\",\"type\":\"input\"}],\"Right\":[{\"id\":\"n\",\"label\":\"-\",\"type\":\"foundation.electrical.electrical\"}],\"Top\":[]}"
  Controlled Temperature Source : fl_lib/Thermal/Thermal Sources/Controlled Temperature Source
      settings: SourceProductBaseCode=PW,SS,VE
  Convective Heat Transfer : fl_lib/Thermal/Thermal Elements/Convective Heat Transfer  area=cell_area m^2  heat_tr_coeff=h_conv W/(m^2 * K)  T_specify=off  T_priority=None  T=0 K  T_nominal_specify=off  T_nominal_unit=K  T_nominal_value=1  Q_specify=off  Q_priority=None  Q=0 W  Q_nominal_specify=off  Q_nominal_unit=W  Q_nominal_value=1
      settings: SourceProductBaseCode=PW,SS,VE
  Em_table : LiBatteryElements_lib/Em_table  C_Table=Capacity_LUT hr*A  Em_Table=Em_LUT V  SOC_Table=SOC_LUT  Temp_Table=Temperature_LUT K  Qinit=Qe_init hr*A
      settings: SourceProductBaseCode=SS  InternalSimscapePortConfiguration="{\"Bottom\":[],\"Left\":[{\"id\":\"p\",\"label\":\"+\",\"type\":\"foundation.electrical.electrical\"},{\"id\":\"C\",\"label\":\"C\",\"type\":\"output\"},{\"id\":\"SOC\",\"label\":\"SOC\",\"type\":\"output\"}],\"Right\":[{\"id\":\"n\",\"label\":\"-\",\"type\":\"foundation.electrical.electrical\"},{\"id\":\"T\",\"label\":\"T\",\"type\":\"input\"}],\"Top\":[]}"
  R0 : LiBatteryElements_lib/R_table  R_Table=R0_LUT Ohm  SOC_Table=SOC_LUT  Temp_Table=Temperature_LUT K
      settings: SourceProductBaseCode=SS  InternalSimscapePortConfiguration="{\"Bottom\":[],\"Left\":[{\"id\":\"p\",\"label\":\"+\",\"type\":\"foundation.electrical.electrical\"},{\"id\":\"T\",\"label\":\"T\",\"type\":\"input\"},{\"id\":\"SOC\",\"label\":\"SOC\",\"type\":\"input\"}],\"Right\":[{\"id\":\"n\",\"label\":\"-\",\"type\":\"foundation.electrical.electrical\"},{\"id\":\"pow\",\"label\":\"POW\",\"type\":\"output\"}],\"Top\":[]}"
  R1 : LiBatteryElements_lib/R_table  R_Table=R1_LUT Ohm  SOC_Table=SOC_LUT  Temp_Table=Temperature_LUT K
      settings: SourceProductBaseCode=SS  InternalSimscapePortConfiguration="{\"Bottom\":[],\"Left\":[{\"id\":\"p\",\"label\":\"+\",\"type\":\"foundation.electrical.electrical\"},{\"id\":\"T\",\"label\":\"T\",\"type\":\"input\"},{\"id\":\"SOC\",\"label\":\"SOC\",\"type\":\"input\"}],\"Right\":[{\"id\":\"n\",\"label\":\"-\",\"type\":\"foundation.electrical.electrical\"},{\"id\":\"pow\",\"label\":\"POW\",\"type\":\"output\"}],\"Top\":[]}"
  R2 : LiBatteryElements_lib/R_table  R_Table=R2_LUT Ohm  SOC_Table=SOC_LUT  Temp_Table=Temperature_LUT K
      settings: SourceProductBaseCode=SS  InternalSimscapePortConfiguration="{\"Bottom\":[],\"Left\":[{\"id\":\"p\",\"label\":\"+\",\"type\":\"foundation.electrical.electrical\"},{\"id\":\"T\",\"label\":\"T\",\"type\":\"input\"},{\"id\":\"SOC\",\"label\":\"SOC\",\"type\":\"input\"}],\"Right\":[{\"id\":\"n\",\"label\":\"-\",\"type\":\"foundation.electrical.electrical\"},{\"id\":\"pow\",\"label\":\"POW\",\"type\":\"output\"}],\"Top\":[]}"
  Simulink-PS Converter1 : nesl_utility/Simulink-PS Converter  PhysicalDomain=network_engine_domain  SubClassName=ps_input  LeftPortType=input  RightPortType=output  PseudoPeriodic=off  Frequencies=[]  NoiseDistribution=none  NoiseParameters=[]  Unit=degC  AffineConversion=on  FilteringAndDerivatives=zero  SimscapeFilterOrder=1  InputFilterTimeConstant=.001  UdotUserProvided=1
      settings: SourceProductBaseCode=SS,PW,VE
  Sum : Subsystem
      mask Display:
      | port_label('RConn',1,'+');
      | port_label('RConn',2,'+');
      | port_label('RConn',3,'+');
  Thermal Model : Subsystem
  Thermal Reference : fl_lib/Thermal/Thermal Elements/Thermal Reference
      settings: SourceProductBaseCode=PW,SS,VE
  + : PMIOPort  Side=Left
  SoC : PMIOPort  Port=2  Side=Right
  Charge : PMIOPort  Port=3  Side=Right
  - : PMIOPort  Port=4  Side=Right
  wires:
  Temp/1 -> Simulink-PS Converter1/1
  connections:
  C1/RConn1 -- R1/RConn1 -- R2/LConn1 -- C2/LConn1
  C1/LConn2 -- R0/LConn2 -- R2/LConn2 -- C2/LConn2 -- Thermal Model/RConn1 -- Em_table/RConn2 -- R1/LConn2
  R0/RConn2 -- Sum/RConn3
  R1/LConn1 -- C1/LConn1 -- Em_table/LConn1
  Convective Heat Transfer/RConn1 -- Thermal Model/LConn2
  R2/RConn1 -- R0/LConn1 -- C2/RConn1
  Sum/RConn2 -- R2/RConn2
  R1/RConn2 -- Sum/RConn1
  SoC/RConn1 -- R0/LConn3 -- C2/LConn3 -- R2/LConn3 -- Em_table/LConn3 -- C1/LConn3 -- R1/LConn3
  Sum/LConn1 -- Thermal Model/LConn1
  Controlled Temperature Source/RConn1 -- Simulink-PS Converter1/RConn1
  Thermal Reference/LConn1 -- Controlled Temperature Source/RConn2
  Controlled Temperature Source/LConn1 -- Convective Heat Transfer/LConn1
  Em_table/RConn1 -- -/RConn1
  R0/RConn1 -- +/RConn1
  Em_table/LConn2 -- Charge/RConn1
